simulink model "Filter"  (R2020a)
settings: Solver=VariableStepAuto  StartTime=0.0  StopTime=10.0  RelTol=1e-3
settings Model: Creator=USER  LastModifiedBy=USER
settings DataIOCC: SaveOutput=off  SaveTime=off

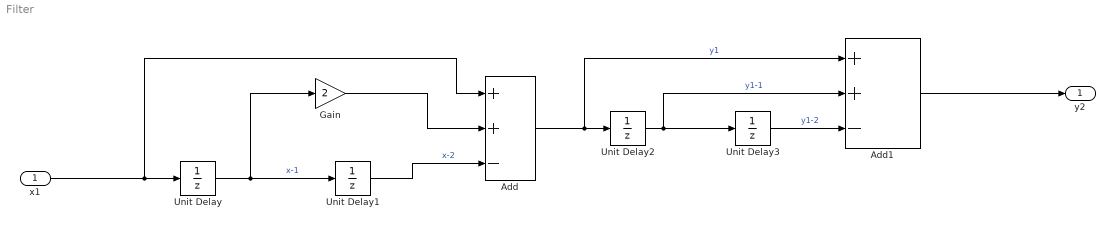
== system Filter ==
  x1 : Inport  OutDataTypeStr=double  PortDimensions=1  SampleTime=[0,1]
  Add : Sum  Inputs=++-
  Add1 : Sum  Inputs=++-
  Gain : Gain  Gain=2
  Unit Delay{,1..3} (4 alike) : UnitDelay  SampleTime=-1  HasFrameUpgradeWarning=on
  y2 : Outport  OutDataTypeStr=double  PortDimensions=1  SampleTime=[0,1]
  wires:
  Unit Delay/1 -> Unit Delay1/1, Gain/1  "x-1"
  Unit Delay2/1 -> Add1/2, Unit Delay3/1  "y1-1"
  x1/1 -> Add/1, Unit Delay/1
  Gain/1 -> Add/2
  Unit Delay3/1 -> Add1/3  "y1-2"
  Add/1 -> Add1/1, Unit Delay2/1  "y1"
  Unit Delay1/1 -> Add/3  "x-2"
  Add1/1 -> y2/1
